simulink model "observer_simulink"  (R2021b)
settings: Solver=VariableStepAuto  StartTime=0.0  StopTime=10  RelTol=1e-3
values from neighbouring files (symbols this model uses):
  A = [0, 0, 0, 1, 0, 0 ... (first row only)    [basic_data.m]    (also in basic_data.mat = [0 0 0 0 -22.4688936865 5 0 0 0 6.5 19.3959496459 -3.6 ... (; lqr.mat = [0 0 0 0 -22.4688936865 5 0 0 0 6.5 19.3959496459 -3.6 ... ()
  B = [0, 0 ... (first row only)    [basic_data.m]    (also in basic_data.mat = [0  0; 0  0; 0  0; 27  11.2; 6.06660129535  -1.63757677119; ; lqr.mat = [0  0; 0  0; 0  0; 27  11.2; 6.06660129535  -1.63757677119; )
  C = [1, 0, 0, 0, 0, 0 ... (first row only)    [basic_data.m]    (also in basic_data.mat = [1 0 0 0 1 0 0 0 1 0 0 0 ... (18 elements, 3x6)]; lqr.mat = [1 0 0 0 1 0 0 0 1 0 0 0 ... (18 elements, 3x6)])
  D = [-2 0 0 ... (first row only)    [observer.m]
  E = double(T*B)    [observer.m]
  G = double([vpa(g11) vpa(g12) vpa(g13); vpa(g21) vpa(g22) vpa(g23); vpa(g31) vpa(g32) vpa(g33)])    [observer.m]
  inv_C_T = inv([C;T])    [observer.m]
  K = real(inv(R)*B'*P)    [ARE.m]    (also in LQR.m = inv(R)*B'*P; Pole_Placement_function.m = h/Wc*S; decoupled.m = F*C_star_star; lqr.mat = [-254.853126299  165.420589601  161.115517614  -14.472900470)
  T = double([1 0 0 vpa(t14) vpa(t15) vpa(t16) ... (first row only)    [observer.m]    (also in pole_placement.m = [C_inv(3, :))
  x_0 = [0.2, -0.1, 0.15, -1, 0.8, 0]'    [basic_data.m]    (also in basic_data.mat = [0.2 -0.1 0.15 -1 0.8 0]; lqr.mat = [0.2 -0.1 0.15 -1 0.8 0])
settings Model: Creator=asus  LastModifiedBy=asus

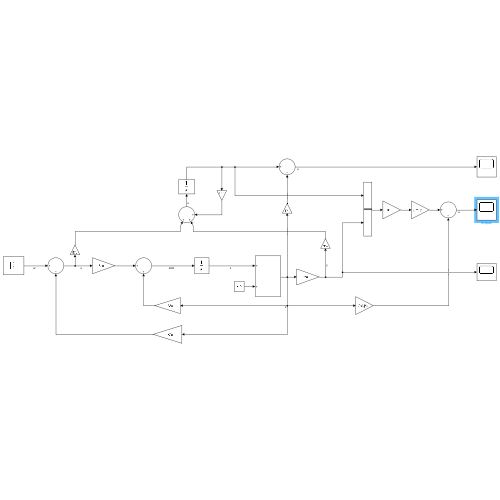
[thumbnail: Simulink's stored preview of the top-level diagram]
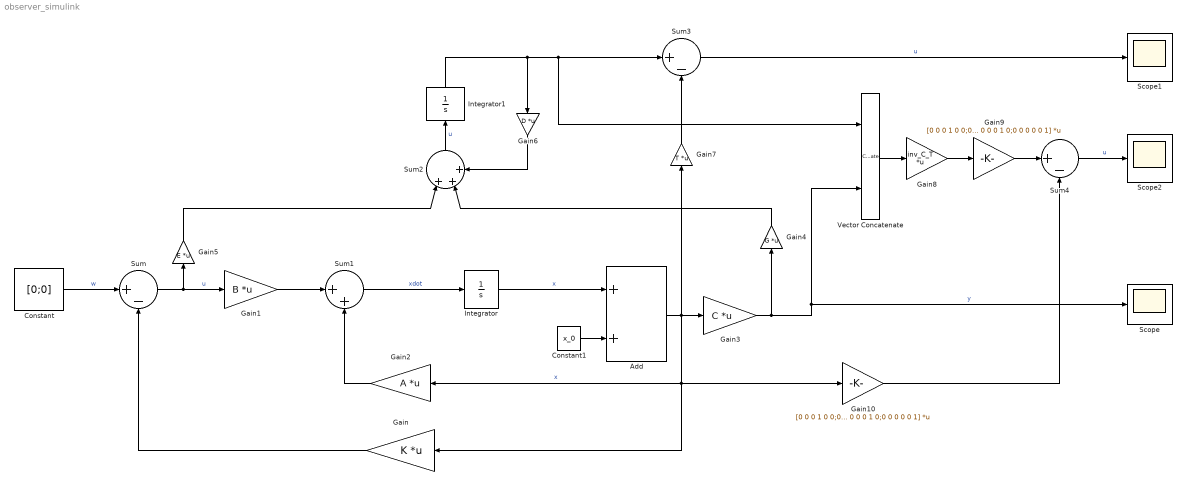
== system observer_simulink ==
  Add : Sum
  Constant : Constant  Value=[0;0]  VectorParams1D=off
  Constant1 : Constant  Value=x_0  VectorParams1D=off
  Gain : Gain  Gain=K  Multiplication=Matrix(K*u)
  Gain1 : Gain  Gain=B  Multiplication=Matrix(K*u)
  Gain10 : Gain  Gain=[0 0 0 1 0 0;0 0 0 0 1 0;0 0 0 0 0 1]  Multiplication=Matrix(K*u)
  Gain2 : Gain  Gain=A  Multiplication=Matrix(K*u)
  Gain3 : Gain  Gain=C  Multiplication=Matrix(K*u)
  Gain4 : Gain  Gain=G  Multiplication=Matrix(K*u)
  Gain5 : Gain  Gain=E  Multiplication=Matrix(K*u)
  Gain6 : Gain  Gain=D  Multiplication=Matrix(K*u)
  Gain7 : Gain  Gain=T  Multiplication=Matrix(K*u)
  Gain8 : Gain  Gain=inv_C_T  Multiplication=Matrix(K*u)
  Gain9 : Gain  Gain=[0 0 0 1 0 0;0 0 0 0 1 0;0 0 0 0 0 1]  Multiplication=Matrix(K*u)
  Integrator : Integrator
  Integrator1 : Integrator
  Scope : Scope
  Scope1 : Scope
  Scope2 : Scope
  Sum : Sum  Inputs=|+-
  Sum1 : Sum  Inputs=|++
  Sum2 : Sum  Inputs=|+++
  Sum3 : Sum  Inputs=|+-
  Sum4 : Sum  Inputs=|+-
  Vector Concatenate : Concatenate
  wires:
  Gain3/1 -> Vector Concatenate/2, Scope/1, Gain4/1  "y"
  Gain2/1 -> Sum1/2
  Gain1/1 -> Sum1/1
  Constant1/1 -> Add/2
  Sum/1 -> Gain1/1, Gain5/1  "u"
  Sum1/1 -> Integrator/1  "xdot"
  Add/1 -> Gain7/1, Gain3/1, Gain2/1, Gain10/1, Gain/1  "x"
  Integrator/1 -> Add/1  "x"
  Constant/1 -> Sum/1  "w"
  Gain/1 -> Sum/2
  Gain5/1 -> Sum2/1
  Gain4/1 -> Sum2/2
  Sum2/1 -> Integrator1/1  "u"
  Gain6/1 -> Sum2/3
  Sum3/1 -> Scope1/1  "u"
  Integrator1/1 -> Vector Concatenate/1, Sum3/1, Gain6/1
  Gain7/1 -> Sum3/2
  Vector Concatenate/1 -> Gain8/1
  Gain8/1 -> Gain9/1
  Gain10/1 -> Sum4/2
  Sum4/1 -> Scope2/1  "u"
  Gain9/1 -> Sum4/1
